simulink model "Demo_M2V5"  (R2015a)
settings: Solver=FixedStepDiscrete  SolverMode=SingleTasking  StartTime=0.0  StopTime=inf  FixedStep=.03  RelTol=1e-3
PostLoadFcn:
  | try,
  | codertarget.arduinobase.registry.setBaudRate(gcs,115200)
  | disp('baud rate set to 115200 for external mode hardware serial')
  | baudrate='set_to_115200'
  | catch
  | disp('baud rate setting not needed in this version')
  | end
libraries: arduinolib x4, MinSegLibrary_M2V5 x4, RASPlib x3
settings Model: SimulationMode=external  ExtModeTrigDuration=2  Creator=Alec  LastModifiedBy=hurstj
settings OptimizationCC: ExpressionDepthLimit=2147483647  OptimizeModelRefInitCode=on  LifeSpan=1
settings DebuggingCC: UnderspecifiedInitializationDetection=Classic  MergeDetectMultiDrivingBlocksExec=none  StateNameClashWarn=warning
settings HardwareCC: ProdBitPerInt=16  ProdBitPerPointer=8  ProdIntDivRoundTo=Zero  ProdEndianess=LittleEndian  ProdWordSize=8  ProdHWDeviceType=Atmel->AVR
settings RTWCC: SystemTargetFile=realtime.tlc  GenerateMakefile=off  TemplateMakefile=realtime.tmf  Description=Real-Time Toolbox  RTWVerbose=off
settings CodeAppCC: CustomSymbolStrType=$N$R$M  InternalIdentifier=Classic
settings ERTTargetCC: CombineOutputUpdateFcns=off  ExtMode=on  ExtModeTransport=3  ExtModeMexArgs=0 7 115200 30  ERTSrcFileBannerTemplate=realtime_code_template.cgt  ERTHdrFileBannerTemplate=realtime_code_template.cgt  ERTDataSrcFileTemplate=realtime_code_template.cgt  ERTDataHdrFileTemplate=realtime_code_template.cgt  ERTCustomFileTemplate=realtime_file_process.tlc

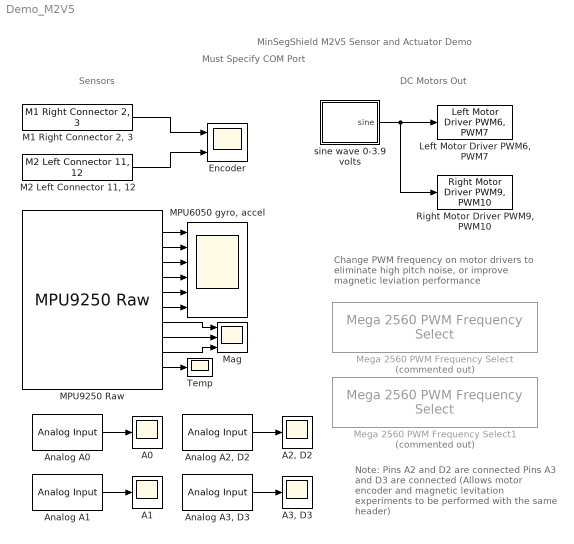
== system Demo_M2V5 ==
  note: Must Specify COM Port
  note: Note: Pins  A2 and D2 are connected
      |          Pins  A3 and D3 are connected
      | (Allows  motor encoder and magnetic
      | levitation experiments to be performed
      | with the same header)
  note: DC Motors Out
  note: Sensors
  note: MinSegShield M2V5 Sensor and Actuator Demo
  note: Change PWM frequency on motor drivers
      | to eliminate high pitch noise, or improve
      | magnetic leviation performance
  A0 : Scope
      settings: YMin=0  YMax=1100  SaveName=ScopeData2
  A1 : Scope
      settings: SaveName=ScopeData3
  "A2, D2" : Scope
      settings: SaveName=ScopeData5
  "A3, D3" : Scope
      settings: SaveName=ScopeData4
  Analog A0 : arduinolib/Analog Input  pinNumber=0  sampleTime=-1  blockPlatform=arduino
  Analog A1 : arduinolib/Analog Input  pinNumber=1  sampleTime=-1  blockPlatform=arduino
  "Analog A2, D2" : arduinolib/Analog Input  pinNumber=2  sampleTime=-1  blockPlatform=arduino
  "Analog A3, D3" : arduinolib/Analog Input  pinNumber=3  sampleTime=-1  blockPlatform=arduino
  Encoder : Scope  NumInputPorts=2
      settings: TimeRange=10  YMin=-7500~-7500  YMax=22500~20000
  "Left Motor Driver PWM6, PWM7" : MinSegLibrary_M2V5/Left Motor Driver PWM6, PWM7  Vsupply=3.9  PWMoffset=0
  "M1 Right Connector 2, 3" : MinSegLibrary_M2V5/M1 Right Connector 2, 3  Encoder=0  PinA=2  PinB=3
  "M2 Left Connector 11, 12" : MinSegLibrary_M2V5/M2 Left Connector 11, 12  Encoder=4  PinA=11  PinB=12
  "MPU6050 gyro, accel" : Scope  NumInputPorts=6
      settings: TimeRange=10  YMin=-15000~-15000~-20000~-10000~-30000~-20000  YMax=15000~7500~25000~10000~40000~15000
  MPU9250 Raw : RASPlib/MPU9250 Raw  SimulateUsing=Code generation
  Mag : Scope  NumInputPorts=3
      settings: TimeRange=10  YMin=-10~-40~-22.5  YMax=12.5~90~0  SaveName=ScopeData7
  Mega 2560 PWM Frequency Select : RASPlib/Mega 2560 PWM Frequency Select  Commented=on  Frequency=32KHz  Timer=4 - pins 6, 7, 8
  Mega 2560 PWM Frequency Select1 : RASPlib/Mega 2560 PWM Frequency Select  Commented=on  Frequency=32KHz  Timer=2 - pins 9, 10
  "Right Motor Driver PWM9, PWM10 " : MinSegLibrary_M2V5/Right Motor Driver PWM9, PWM10   Vsupply=3.9  PWMoffset=0
  Temp : Scope
      settings: TimeRange=30  YMin=1500  YMax=1650  SaveName=ScopeData9
  sine wave 0-3.9 volts : Subsystem
  wires:
  sine wave 0-3.9 volts/1(sine) -> "Right Motor Driver PWM9, PWM10 "/1, "Left Motor Driver PWM6, PWM7"/1
  "M1 Right Connector 2, 3"/1 -> Encoder/1
  "M2 Left Connector 11, 12"/1 -> Encoder/2
  Analog A0/1 -> A0/1
  Analog A1/1 -> A1/1
  "Analog A2, D2"/1 -> "A2, D2"/1
  MPU9250 Raw/2 -> "MPU6050 gyro, accel"/2
  MPU9250 Raw/3 -> "MPU6050 gyro, accel"/3
  MPU9250 Raw/4 -> "MPU6050 gyro, accel"/4
  MPU9250 Raw/5 -> "MPU6050 gyro, accel"/5
  MPU9250 Raw/6 -> "MPU6050 gyro, accel"/6
  MPU9250 Raw/7 -> Mag/1
  MPU9250 Raw/8 -> Mag/2
  MPU9250 Raw/9 -> Mag/3
  MPU9250 Raw/10 -> Temp/1
  MPU9250 Raw/1 -> "MPU6050 gyro, accel"/1
  "Analog A3, D3"/1 -> "A3, D3"/1

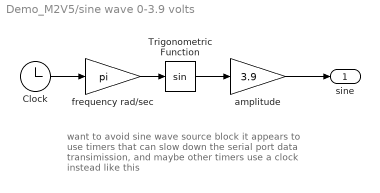
== system Demo_M2V5/sine wave 0-3.9 volts ==
  note: want to avoid sine wave source block
      | it appears to use timers that can slow down the
      | serial port data transimission, and maybe
      | other timers
      |
      | use a clock instead like this
  Clock : Clock
  Trigonometric Function : Trigonometry
  amplitude : Gain  Gain=3.9
  frequency rad/sec : Gain  Gain=pi
  sine : Outport
  wires:
  Clock/1 -> frequency rad/sec/1
  Trigonometric Function/1 -> amplitude/1
  frequency rad/sec/1 -> Trigonometric Function/1
  amplitude/1 -> sine/1
